simulink model "VDC"  (R2022a)
settings: Solver=VariableStepAuto  StartTime=0.0  StopTime=10.0  RelTol=1e-3
values from neighbouring files (symbols this model uses):
  Bm = 3.2106*10^-4    (= 0.00032106)    [par.m]
  Bm_hat = 2*10^-4    (= 0.0002)    [par.m]
  Jm = 1.9171*10^-4    (= 0.00019171)    [par.m]
  Jm_hat = 1.5*10^-4    (= 0.00015)    [par.m]
  K1 = 10    [par.m]
  K2 = 1    [par.m]
  Ki = 0.02    [par.m]
  Kp = 5.0    (= 5)    [par.m]
  Noise = 0.001    [par.m]
  Td = 10    [par.m]
libraries: simulink x1
settings Model: Creator=rock8  LastModifiedBy=rock8

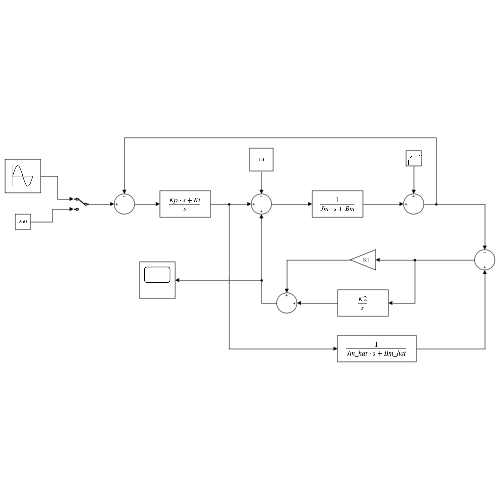
[thumbnail: Simulink's stored preview of the top-level diagram]
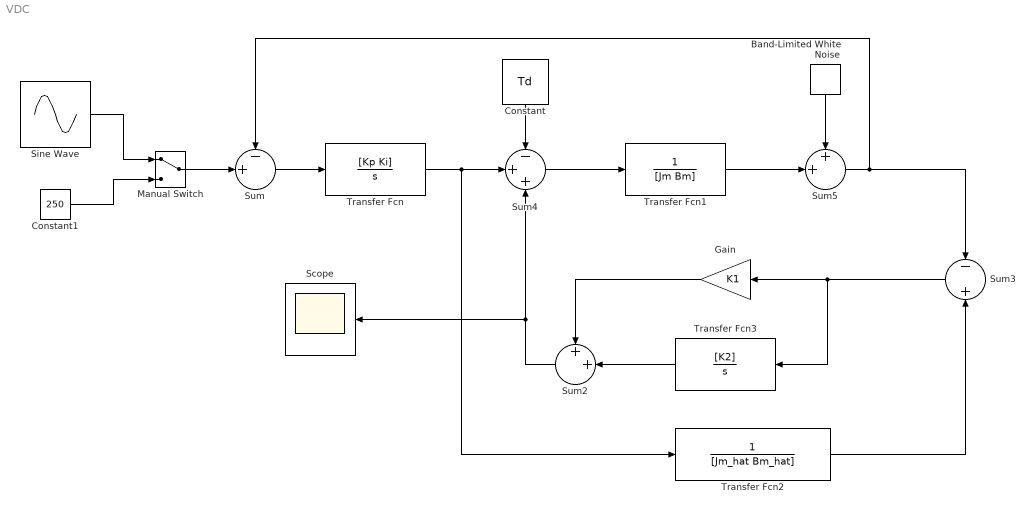
== system VDC ==
  Band-Limited White Noise : simulink/Sources/Band-Limited White Noise  Cov=[Noise]  Ts=0.1  seed=[23341]
  Constant : Constant  Value=Td
  Constant1 : Constant  Value=250
  Gain : Gain  Gain=K1
  Manual Switch : ManualSwitch
  Scope : Scope
  Sine Wave : Sin  Amplitude=250  SampleTime=0
  Sum : Sum  Inputs=-+|
  Sum2 : Sum  Inputs=++|
  Sum3 : Sum  Inputs=-|+
  Sum4 : Sum  Inputs=-++
  Sum5 : Sum  Inputs=++|
  Transfer Fcn : TransferFcn  Numerator=[Kp Ki]  Denominator=[1 0]
  Transfer Fcn1 : TransferFcn  Denominator=[Jm Bm]
  Transfer Fcn2 : TransferFcn  Denominator=[Jm_hat Bm_hat]
  Transfer Fcn3 : TransferFcn  Numerator=[K2]  Denominator=[1 0]
  wires:
  Sum/1 -> Transfer Fcn/1
  Sum4/1 -> Transfer Fcn1/1
  Sum3/1 -> Transfer Fcn3/1, Gain/1
  Transfer Fcn2/1 -> Sum3/2
  Transfer Fcn3/1 -> Sum2/2
  Gain/1 -> Sum2/1
  Transfer Fcn/1 -> Transfer Fcn2/1, Sum4/2
  Constant/1 -> Sum4/1
  Transfer Fcn1/1 -> Sum5/2
  Sum5/1 -> Sum3/1, Sum/1
  Band-Limited White Noise/1 -> Sum5/1
  Sum2/1 -> Sum4/3, Scope/1
  Manual Switch/1 -> Sum/2
  Sine Wave/1 -> Manual Switch/1
  Constant1/1 -> Manual Switch/2
